simulink model "control_system_small"  (R2020b)
settings: Solver=ode23t  StartTime=0.0  StopTime=5.5  RelTol=1e-3  AbsTol=1e-07
model workspace (MAT data in the model file):
  l = 2
  wfb = [0; 0; 0]
undefined symbols (not defined in the file): dt
libraries: lib_beam x25
settings Model: Creator=hao  LastModifiedBy=hao
settings DebuggingCC: UnconnectedInputMsg=none  UnconnectedOutputMsg=none  UnderSpecifiedDimensionMsg=warning

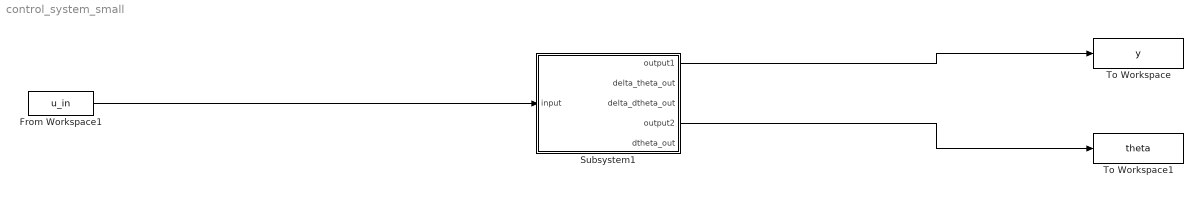
== system control_system_small ==
  From Workspace1 : FromWorkspace  VariableName=u_in  SampleTime=dt
  Subsystem1 : Subsystem
  To Workspace : ToWorkspace  VariableName=y  SaveFormat=Timeseries  SampleTime=dt
  To Workspace1 : ToWorkspace  VariableName=theta  SaveFormat=Timeseries  SampleTime=dt
  wires:
  From Workspace1/1 -> Subsystem1/1(input)
  Subsystem1/1(output1) -> To Workspace/1
  Subsystem1/4(output2) -> To Workspace1/1

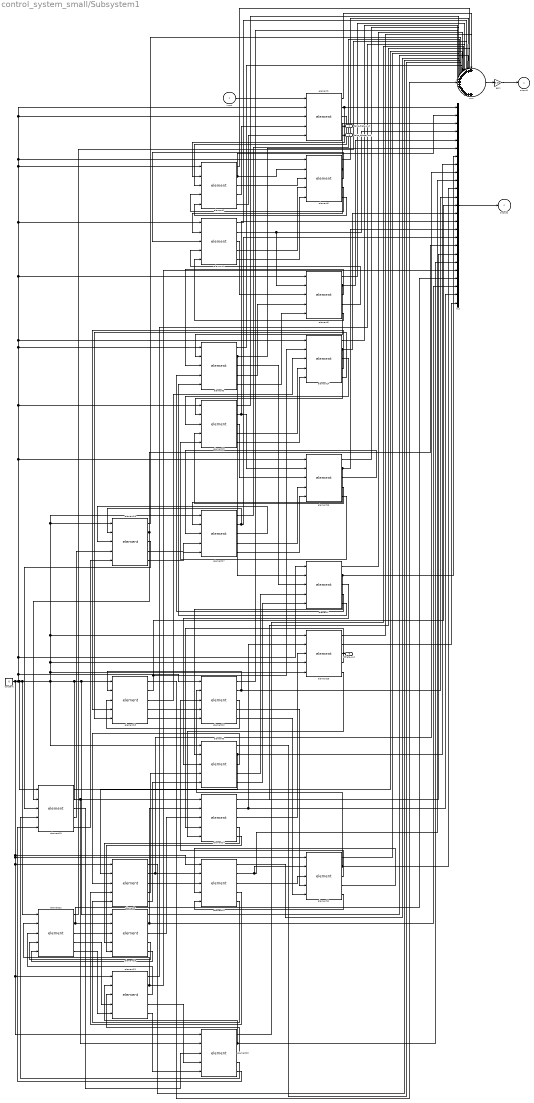
== system control_system_small/Subsystem1 ==
  input : Inport
  bus : BusCreator  Inputs=25
  constant : Constant  Value=0
  element{1..25} (25 alike) : lib_beam/element  IA=0.005  k1=5  k2=1000  k3=10000  b=30  ElementLength=0
  gain : Gain  Gain=0.03
  sum : Sum  Inputs=25
  output1 : Outport
  delta_theta_out : Outport  Port=2
  delta_dtheta_out : Outport  Port=3
  output2 : Outport  Port=4
  dtheta_out : Outport  Port=5
  wires:
  element23/5 -> element22/5
  element3/4 -> element2/4
  element18/1 -> sum/18
  element2/3 -> element3/3
  element25/5 -> element24/5
  element20/4 -> element19/4
  element20/3 -> element21/3
  element8/5 -> element7/5
  element22/4 -> element21/4
  element23/3 -> element24/3
  element13/3 -> element14/3
  element11/2 -> bus/11, element12/2
  element10/2 -> bus/10, element11/2
  element18/4 -> element17/4
  element6/4 -> element5/4
  element24/4 -> element23/4
  element2/1 -> sum/2
  element5/1 -> sum/5
  element2/4 -> element1/4
  element23/1 -> sum/23
  element9/5 -> element8/5
  element3/3 -> element4/3
  element20/1 -> sum/20
  element24/3 -> element25/3
  element1/2 -> bus/1, element2/2
  element9/4 -> element8/4
  element8/3 -> element9/3
  element4/1 -> sum/4
  element15/4 -> element14/4
  element15/3 -> element16/3
  element22/5 -> element21/5
  element21/5 -> element20/5
  element15/2 -> bus/15, element16/2
  element23/4 -> element22/4
  element7/5 -> element6/5
  gain/1 -> output1/1
  element17/5 -> element16/5
  element4/2 -> bus/4, element5/2
  element7/2 -> bus/7, element8/2
  element21/4 -> element20/4
  element19/5 -> element18/5
  element11/5 -> element10/5
  element6/3 -> element7/3
  element3/2 -> bus/3, element4/2
  element12/4 -> element11/4
  element20/5 -> element19/5
  element16/2 -> bus/16, element17/2
  element9/2 -> bus/9, element10/2
  element22/3 -> element23/3
  element19/1 -> sum/19
  element21/3 -> element22/3
  bus/1 -> output2/1
  element11/3 -> element12/3
  element17/1 -> sum/17
  element16/3 -> element17/3
  element18/2 -> bus/18, element19/2
  element2/5 -> element1/5
  element16/5 -> element15/5
  element24/1 -> sum/24
  element7/1 -> sum/7
  element5/4 -> element4/4
  sum/1 -> gain/1
  element25/3 -> dtheta_out/1
  element14/5 -> element13/5
  constant/1 -> element20/1, element21/1, element9/1, element11/1, element10/1, element13/1, element23/1, element24/1, element17/1, element18/1, element25/1, element25/4, element25/5, element8/1, element22/1, element19/1, element1/2, element1/3, element3/1, element2/1, element4/1, element5/1, element14/1, element6/1, element15/1, element16/1, element7/1, element12/1
  element12/1 -> sum/12
  element18/5 -> element17/5
  element7/3 -> element8/3
  element15/5 -> element14/5
  element5/5 -> element4/5
  element1/4 -> delta_theta_out/1
  element15/1 -> sum/15
  element14/1 -> sum/14
  element8/4 -> element7/4
  element13/5 -> element12/5
  element21/2 -> bus/21, element22/2
  element14/4 -> element13/4
  element8/2 -> bus/8, element9/2
  element3/1 -> sum/3
  element16/1 -> sum/16
  element6/2 -> bus/6, element7/2
  element13/4 -> element12/4
  element22/2 -> bus/22, element23/2
  element19/2 -> bus/19, element20/2
  element1/5 -> delta_dtheta_out/1
  element2/2 -> bus/2, element3/2
  element25/2 -> bus/25
  element25/4 -> element24/4
  element21/1 -> sum/21
  element12/5 -> element11/5
  element6/1 -> sum/6
  element11/1 -> sum/11
  element25/1 -> sum/25
  element10/5 -> element9/5
  element1/3 -> element2/3
  element17/2 -> bus/17, element18/2
  element1/1 -> sum/1
  input/1 -> element1/1
  element11/4 -> element10/4
  element4/3 -> element5/3
  element6/5 -> element5/5
  element10/3 -> element11/3
  element13/1 -> sum/13
  element24/2 -> bus/24, element25/2
  element12/3 -> element13/3
  element24/5 -> element23/5
  element9/3 -> element10/3
  element4/4 -> element3/4
  element13/2 -> bus/13, element14/2
  element10/4 -> element9/4
  element4/5 -> element3/5
  element17/3 -> element18/3
  element5/3 -> element6/3
  element20/2 -> bus/20, element21/2
  element23/2 -> bus/23, element24/2
  element19/3 -> element20/3
  element12/2 -> bus/12, element13/2
  element14/3 -> element15/3
  element9/1 -> sum/9
  element8/1 -> sum/8
  element5/2 -> bus/5, element6/2
  element17/4 -> element16/4
  element18/3 -> element19/3
  element14/2 -> bus/14, element15/2
  element19/4 -> element18/4
  element16/4 -> element15/4
  element22/1 -> sum/22
  element7/4 -> element6/4
  element10/1 -> sum/10
  element3/5 -> element2/5
